simulink model "Relational_Operator_with_Stepinput"  (R2023a)
settings: Solver=FixedStepAuto  StartTime=0.0  StopTime=10  FixedStep=1e-3  RelTol=1e-3
settings Model: Creator=Mass  LastModifiedBy=Mass

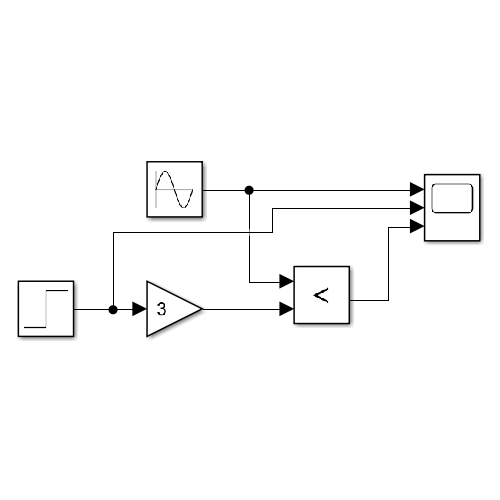
[thumbnail: Simulink's stored preview of the top-level diagram]
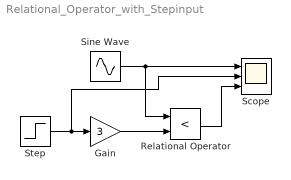
== system Relational_Operator_with_Stepinput ==
  Gain : Gain  Gain=3
  Relational Operator : RelationalOperator  Operator=<  OutDataTypeStr=boolean  RndMeth=Simplest  InputSameDT=off
  Scope : Scope  NumInputPorts=3
  Sine Wave : Sin  Frequency=2*pi  SampleTime=0
  Step : Step  Time=2  SampleTime=0
  wires:
  Sine Wave/1 -> Relational Operator/1, Scope/1
  Step/1 -> Scope/2, Gain/1
  Gain/1 -> Relational Operator/2
  Relational Operator/1 -> Scope/3
